simulink model "goto_from_test_tmp"  (Simulink 8.3)
settings: Solver=ode45  StartTime=0.0  StopTime=10.0  RelTol=1e-3
settings Model: Creator=arnaud  LastModifiedBy=hbourbou
settings DataIOCC: SaveFormat=Structure  SignalLoggingSaveFormat=Dataset
settings DebuggingCC: UnderspecifiedInitializationDetection=Simplified  MergeDetectMultiDrivingBlocksExec=error  FrameProcessingCompatibilityMsg=error  StateNameClashWarn=none
settings GRTTargetCC: CombineOutputUpdateFcns=on  GRTInterface=off

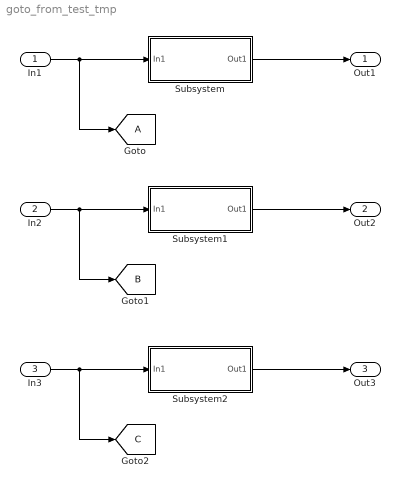
== system goto_from_test_tmp ==
  In1 : Inport  OutDataTypeStr=double
  In2 : Inport  Port=2  OutDataTypeStr=int32  PortDimensions=2
  In3 : Inport  Port=3  OutDataTypeStr=boolean  PortDimensions=[2 3]
  Subsystem : Subsystem
  Subsystem1 : Subsystem
  Subsystem2 : Subsystem
  Out1 : Outport
  Out2 : Outport  Port=2
  Out3 : Outport  Port=3
  tag scope: A=global, B=global, C=global
  wires:
  Subsystem/1(Out1) -> Out1/1
  In1/1 -> [A], Subsystem/1(In1)
  Subsystem1/1(Out1) -> Out2/1
  In2/1 -> [B], Subsystem1/1(In1)
  Subsystem2/1(Out1) -> Out3/1
  In3/1 -> [C], Subsystem2/1(In1)

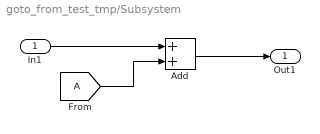
== system goto_from_test_tmp/Subsystem ==
  In1 : Inport
  Add : Sum
  Out1 : Outport
  wires:
  [A] -> Add/2
  In1/1 -> Add/1
  Add/1 -> Out1/1

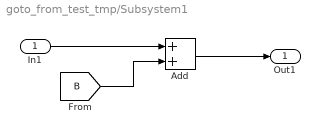
== system goto_from_test_tmp/Subsystem1 ==
  In1 : Inport
  Add : Sum
  Out1 : Outport
  wires:
  [B] -> Add/2
  In1/1 -> Add/1
  Add/1 -> Out1/1

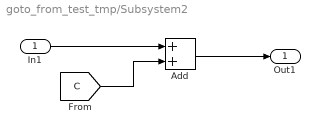
== system goto_from_test_tmp/Subsystem2 ==
  In1 : Inport
  Add : Sum
  Out1 : Outport
  wires:
  [C] -> Add/2
  In1/1 -> Add/1
  Add/1 -> Out1/1
